simulink model "lab2_part2"  (R2025b)
settings: Solver=VariableStepAuto  StartTime=0.0  StopTime=30.0  RelTol=1e-10  AbsTol=1e-10
values from neighbouring files (symbols this model uses):
  A = [0 1; 0 -alpha_2/M]    [lab2.m]
  Actrl = A + B*K - L*C    [lab2.m]
  B = [0; alpha_1/M]    [lab2.m]
  Bctrl = [L -B*K]    [lab2.m]
  C = [1 0]    [lab2.m]
  Cctrl = K    [lab2.m]
  Dctrl = [0 -K]    [lab2.m]

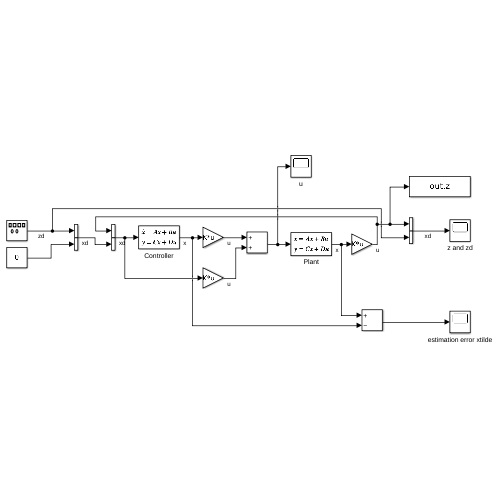
[thumbnail: Simulink's stored preview of the top-level diagram]
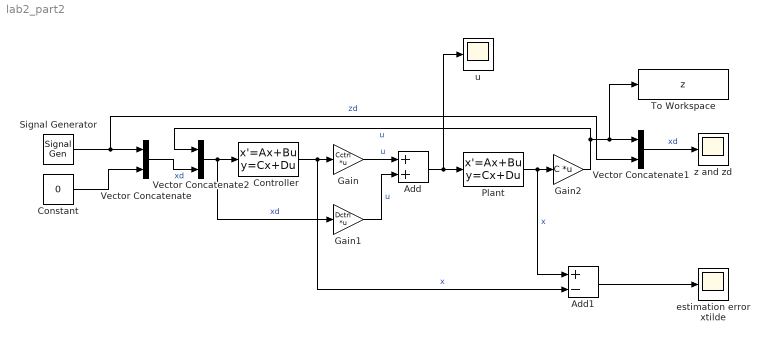
== system lab2_part2 ==
  Add : Sum
  Add1 : Sum  Inputs=+-
  Constant : Constant  Value=0
  Controller : StateSpace  A=Actrl  B=Bctrl  C=eye(2)  D=zeros(2,3)  InitialCondition=0
  Gain : Gain  Gain=Cctrl  Multiplication=Matrix(K*u)
  Gain1 : Gain  Gain=Dctrl  Multiplication=Matrix(K*u)
  Gain2 : Gain  Gain=C  Multiplication=Matrix(K*u)
  Plant : StateSpace  A=A  B=B  C=eye(2)  D=zeros(2,1)  InitialCondition=0
  Signal Generator : SignalGenerator  WaveForm=square  Amplitude=0.03  Frequency=0.1
  To Workspace : ToWorkspace  VariableName=z  SaveFormat=Timeseries  SampleTime=-1
  Vector Concatenate : Concatenate
  Vector Concatenate1 : Concatenate
  Vector Concatenate2 : Concatenate
  estimation error xtilde : Scope
      settings: ActiveDisplayYMinimum=-5.72963823064241E-14  ActiveDisplayYMaximum=4.2703617693575913E-14
  u : Scope
      settings: ActiveDisplayYMinimum=-10.390527611429157  ActiveDisplayYMaximum=5.2240908278154929  DataLoggingVariableName=ScopeData2
  z and zd : Scope
      settings: ActiveDisplayYMinimum=-0.060685473335787866  ActiveDisplayYMaximum=0.070226710404598131
  wires:
  Signal Generator/1 -> Vector Concatenate1/2, Vector Concatenate/1  "zd"
  Constant/1 -> Vector Concatenate/2
  Vector Concatenate1/1 -> z and zd/1  "xd"
  Vector Concatenate/1 -> Vector Concatenate2/2  "xd"
  Vector Concatenate2/1 -> Gain1/1, Controller/1  "xd"
  Controller/1 -> Add1/2, Gain/1  "x"
  Add/1 -> u/1, Plant/1
  Gain/1 -> Add/1  "u"
  Gain1/1 -> Add/2  "u"
  Plant/1 -> Add1/1, Gain2/1  "x"
  Gain2/1 -> To Workspace/1, Vector Concatenate1/1, Vector Concatenate2/1  "u"
  Add1/1 -> estimation error xtilde/1
